simulink model "KalSim"  (Simulink 8.2)
settings: Solver=FixedStepDiscrete  StartTime=0.0  StopTime=16  FixedStep=0.005  RelTol=1e-3
PostLoadFcn:
  | , if any(exist('dsrtsu_mdlpostloadfcn', 'file') == [2, 3, 6]), try dsrtsu_mdlpostloadfcn('Execute', bdroot); catch fprintf('Error in PostLoadFcn (dsrtsu_mdlpostloadfcn) for model "%s":\n %s\n', bdroot, lasterr); end, end,
values from neighbouring files (symbols this model uses):
  C_TASK_5MS_S = (	C_TICK_TIME_S      	)    [hcu_local_hdr.m]
  FALSE = boolean( 0 )    [hcu_local_hdr.m]
  TRUE = boolean( 1 )    [hcu_local_hdr.m]
undefined symbols (not defined in the file or in its folder): A_TTC, B_TTC, C_TTC, divide, Gamma_TTC, hcu_lib, KTTC_KalmanFilterCalRate_s, Q_TTC, R_TTC_Position, R_TTC_RelAccel, R_TTC_RelVelocity
libraries: dspmtrx3 x3, simulink x1, dspinverses x1
settings Model: DSRTSU_INTERNAL_RTI_VER=460  DSRTSU_INTERNAL_RTI_TYPE=rti1401  RTICANMMDATA=struct('GeneralSetupData',struct('modelroot','D:\HAITEC\SVN\trunk\ADAS_Softwares\HTDragon\software\sw_development\arch','generalsettings',struct('filesettings',struct('destfolder',struct('Name','RTICANMM_FILES','Check',1),'buildfolder',struct('Name','.','Check',1),'AbsDestfolder',struct('Name','D:\HAITEC\SVN\trunk\ADAS_Softwares\HTDragon\software\sw_development\arch\RTICANMM_FILES'),'AbsBuildfolder',struct('Name','D:\HAITEC\SVN\trunk\ADAS_Softwares\HTDragon\software\sw_development\arch'))),'options',struct('addpaths',1,'rmpaths',1,'addtrcexclusion',logical(1),'cannavigator',struct('checkmonitoring',0),'show_usrtrc',0,'use_usrtrc',0),'advanced',struct('options',[1 1 1 1 1 1 1 1 1 1 1 1 1 1 1 1 1 1 1 1 1 1 1 1 1 1 1 1 1 1 1 1 1 1 1 1 1 1 1 1 1 1 1 1 1 1 1 1 1 1 1 1 1 1 1 1 1 1 1 1 1 1 1 1 1 1 1 1 1 1 1 1 1 1 1 1 1 1 1 1 1 1 1 1 1 1 1 1 1 1 1 1 1 1 1 1 1 1 1 1]),'MPSetup',{{}},'modelname','KalSim','block','KalSim'))  DSRTSU_INTERNAL_RTIFPGA=50  Creator=14014  LastModifiedBy=14014  BufferReuse=off
settings DataIOCC: SignalLoggingSaveFormat=Dataset
settings OptimizationCC: BlockReduction=off  OptimizeBlockIOStorage=off  BufferReuse=off  ExpressionFolding=off  ExpressionDepthLimit=128  LocalBlockOutputs=off
settings DebuggingCC: InheritedTsInSrcMsg=none  ParameterPrecisionLossMsg=none  FcnCallInpInsideContextMsg=EnableAllAsError  StateNameClashWarn=none
settings HardwareCC: ProdIntDivRoundTo=Zero  ProdEndianess=BigEndian  ProdHWDeviceType=Generic->Custom  TargetIntDivRoundTo=Zero  TargetEndianess=BigEndian  TargetHWDeviceType=Generic->Custom
settings RTWCC: SystemTargetFile=rti1401.tlc  MakeCommand=make_rti  TemplateMakefile=rti1401.tmf  Description=dSPACE DS1401 Hardware Platform  ProcessScript=rti1401_make_rtw_hook
settings STFCustomTargetCC: CodeReplacementLibrary=ANSI_C  ParMdlRefBuildCompliant=on  GeneratePreprocessorConditionals=Disable all  MatFileLogging=on  SystemTargetFile=rti1401.tlc
settings GRTTargetCC: CompOptLevelCompliant=off  ConcurrentExecutionCompliant=off  ExtModeMexFile=noextcomm
settings CustomProperty: DataType=RTWOptions_EnumType_C__Program Files_dSPACE RCPHIL 2015-A_MATLAB_RTI_RTI1401_TLC_rti1401_1InitialSimState  Value=RUN
settings EnumStrPairs: String=RUN

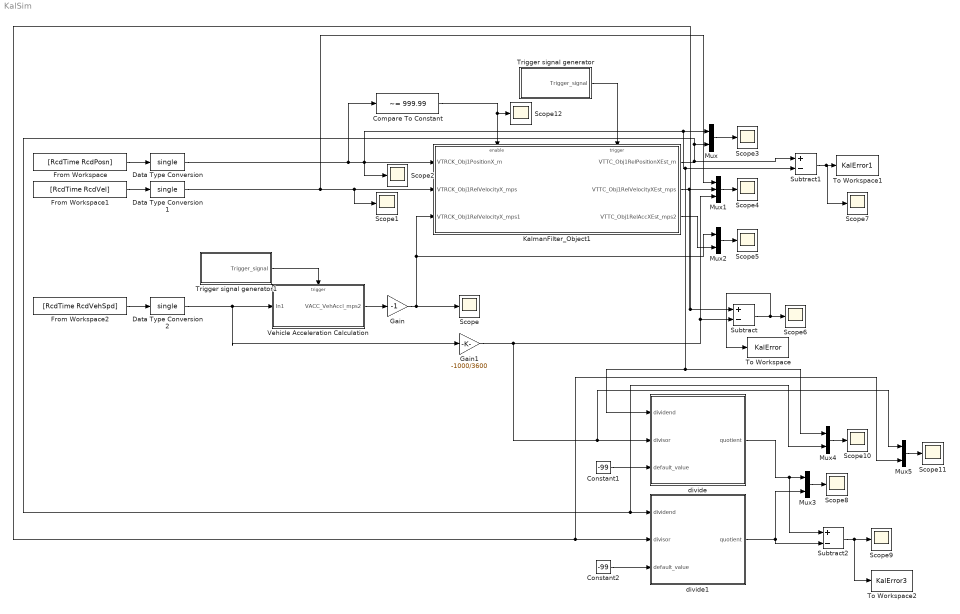
== system KalSim ==
  Compare To Constant : simulink/Logic and Bit Operations/Compare To Constant  relop=~=  const=999.99  OutDataTypeStr=boolean
  Constant1 : Constant  Value=-99  OutDataTypeStr=single
  Constant2 : Constant  Value=-99  OutDataTypeStr=single
  Data Type Conversion : DataTypeConversion  OutDataTypeStr=single
  Data Type Conversion1 : DataTypeConversion  OutDataTypeStr=single
  Data Type Conversion2 : DataTypeConversion  OutDataTypeStr=single
  From Workspace : FromWorkspace  VariableName=[RcdTime RcdPosn]
  From Workspace1 : FromWorkspace  VariableName=[RcdTime RcdVel]
  From Workspace2 : FromWorkspace  VariableName=[RcdTime RcdVehSpd]
  Gain : Gain  Gain=-1
  Gain1 : Gain  Gain=-1000/3600
  KalmanFilter_Object1 : Subsystem
  Mux{,2..5} (5 alike) : Mux  Inputs=2
  Mux1 : Mux  Inputs=3
  Scope{,1..12} (13 alike) : Scope
      Scope10 settings: SaveName=ScopeData7
      Scope11 settings: SaveName=ScopeData8
      Scope12 settings: SaveName=ScopeData9
      Scope2 settings: SaveName=ScopeData2
      Scope3 settings: SaveName=ScopeData3
      Scope4 settings: SaveName=ScopeData4
      Scope5 settings: SaveName=ScopeData5
      Scope6 settings: SaveName=KalError
      Scope7 settings: SaveName=KalError2
      Scope8 settings: SaveName=ScopeData6
      Scope9 settings: SaveName=KalError3
  Subtract : Sum  Inputs=+-
  Subtract1 : Sum  Inputs=+-
  Subtract2 : Sum  Inputs=+-
  To Workspace : ToWorkspace  VariableName=KalError  SampleTime=-1
  To Workspace1 : ToWorkspace  VariableName=KalError1  SampleTime=-1
  To Workspace2 : ToWorkspace  VariableName=KalError3  SampleTime=-1
  Trigger signal generator : Subsystem  TreatAsAtomicUnit=on
  Trigger signal generator1 : Subsystem  TreatAsAtomicUnit=on
  Vehicle Acceleration Calculation : Subsystem
  divide : Subsystem  AncestorBlock=hcu_lib/divide  RTWFcnName=divide_safe  RTWFileName=HCU_LIB  mask(divide){}
      mask help: Performs a division operation. If the divisor is found to be between -0.00001 and +0.00001 then a failsafe value is passed to the output.
      settings: RTWFcnNameOpts=User specified  RTWFileNameOpts=User specified
      mask Display: disp('Divide');
  divide1 : Subsystem  AncestorBlock=hcu_lib/divide  RTWFcnName=divide_safe  RTWFileName=HCU_LIB  mask(divide){}
      mask help: Performs a division operation. If the divisor is found to be between -0.00001 and +0.00001 then a failsafe value is passed to the output.
      settings: RTWFcnNameOpts=User specified  RTWFileNameOpts=User specified
      mask Display: disp('Divide');
  wires:
  From Workspace/1 -> Data Type Conversion/1
  From Workspace1/1 -> Data Type Conversion1/1
  Trigger signal generator/1(Trigger_signal) -> KalmanFilter_Object1/Trigger
  Compare To Constant/1 -> Scope12/1, KalmanFilter_Object1/Enable
  From Workspace2/1 -> Data Type Conversion2/1
  Data Type Conversion/1 -> Compare To Constant/1, divide/1(dividend), Mux4/1, Subtract1/2, Mux/1, Scope2/1, KalmanFilter_Object1/1(VTRCK_Obj1PositionX_m)
  Data Type Conversion1/1 -> Mux1/1, Scope1/1, KalmanFilter_Object1/2(VTRCK_Obj1RelVelocityX_mps)
  Trigger signal generator1/1(Trigger_signal) -> Vehicle Acceleration Calculation/Trigger
  Data Type Conversion2/1 -> Gain1/1, Vehicle Acceleration Calculation/1(In1)
  Vehicle Acceleration Calculation/1(VACC_VehAccl_mps2) -> Gain/1
  Gain/1 -> Scope/1, KalmanFilter_Object1/3(VTRCK_Obj1RelVelocityX_mps1), Mux2/1
  KalmanFilter_Object1/1(VTTC_Obj1RelPositionXEst_m) -> Mux4/2, divide1/1(dividend), Mux/2, Subtract1/1
  Mux/1 -> Scope3/1
  KalmanFilter_Object1/2(VTTC_Obj1RelVelocityXEst_mps) -> Mux5/2, divide1/2(divisor), Subtract/1, Mux1/2
  Mux1/1 -> Scope4/1
  Mux2/1 -> Scope5/1
  KalmanFilter_Object1/3(VTTC_Obj1RelAccXEst_mps2) -> Mux2/2
  Gain1/1 -> Mux5/1, divide/2(divisor), Subtract/2, Mux1/3
  Subtract/1 -> To Workspace/1, Scope6/1
  Subtract1/1 -> Scope7/1, To Workspace1/1
  Constant1/1 -> divide/3(default_value)
  Constant2/1 -> divide1/3(default_value)
  Mux3/1 -> Scope8/1
  divide/1(quotient) -> Subtract2/1, Mux3/1
  divide1/1(quotient) -> Subtract2/2, Mux3/2
  Subtract2/1 -> To Workspace2/1, Scope9/1
  Mux4/1 -> Scope10/1
  Mux5/1 -> Scope11/1

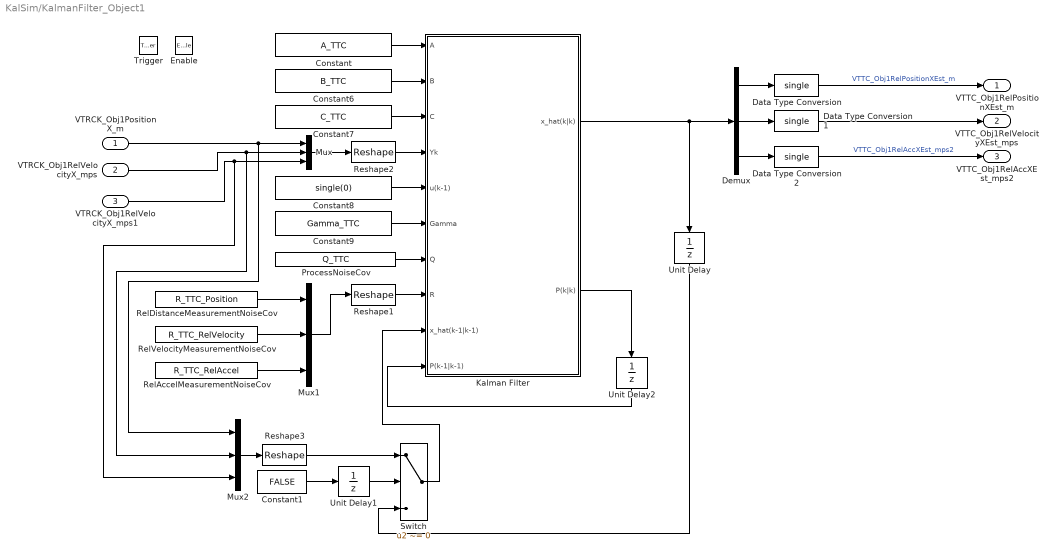
== system KalSim/KalmanFilter_Object1 ==
  VTRCK_Obj1PositionX_m : Inport
  VTRCK_Obj1RelVelocityX_mps : Inport  Port=2
  VTRCK_Obj1RelVelocityX_mps1 : Inport  Port=3
  Enable : EnablePort  StatesWhenEnabling=reset
  Trigger : TriggerPort  PortDimensions=1
  Constant : Constant  Value=A_TTC
  Constant1 : Constant  Value=FALSE
  Constant6 : Constant  Value=B_TTC
  Constant7 : Constant  Value=C_TTC
  Constant8 : Constant  Value=single(0)
  Constant9 : Constant  Value=Gamma_TTC
  Data Type Conversion : DataTypeConversion  OutDataTypeStr=single
  Data Type Conversion1 : DataTypeConversion  OutDataTypeStr=single
  Data Type Conversion2 : DataTypeConversion  OutDataTypeStr=single
  Demux : Demux  Outputs=3
  Kalman Filter : Subsystem
  Mux : Mux  Inputs=3
  Mux1 : Mux  Inputs=3
  Mux2 : Mux  Inputs=3
  ProcessNoiseCov : Constant  Value=Q_TTC
  RelAccelMeasurementNoiseCov : Constant  Value=R_TTC_RelAccel  OutDataTypeStr=single
  RelDistanceMeasurementNoiseCov : Constant  Value=R_TTC_Position  OutDataTypeStr=single
  RelVelocityMeasurementNoiseCov : Constant  Value=R_TTC_RelVelocity  OutDataTypeStr=single
  Reshape1 : Reshape  OutputDimensionality=Customize  OutputDimensions=[3,3]
  Reshape2 : Reshape  OutputDimensionality=Customize  OutputDimensions=[3,1]
  Reshape3 : Reshape  OutputDimensionality=Customize  OutputDimensions=[3,1]
  Switch : Switch  Criteria=u2 ~= 0
  Unit Delay : UnitDelay  InitialCondition=single([0;0;0])  SampleTime=-1
  Unit Delay1 : UnitDelay  InitialCondition=TRUE  SampleTime=-1
  Unit Delay2 : UnitDelay  InitialCondition=single(eye(3,3))  SampleTime=-1
  VTTC_Obj1RelPositionXEst_m : Outport  OutputWhenDisabled=reset  InitialOutput=[0]
  VTTC_Obj1RelVelocityXEst_mps : Outport  Port=2  OutputWhenDisabled=reset  InitialOutput=[0]
  VTTC_Obj1RelAccXEst_mps2 : Outport  Port=3  OutputWhenDisabled=reset  InitialOutput=[0]
  wires:
  Data Type Conversion2/1 -> VTTC_Obj1RelAccXEst_mps2/1  "VTTC_Obj1RelAccXEst_mps2"
  Data Type Conversion1/1 -> VTTC_Obj1RelVelocityXEst_mps/1
  Data Type Conversion/1 -> VTTC_Obj1RelPositionXEst_m/1  "VTTC_Obj1RelPositionXEst_m"
  Kalman Filter/2(P(k|k)) -> Unit Delay2/1
  Unit Delay2/1 -> Kalman Filter/10(P(k-1|k-1))
  Kalman Filter/1(x_hat(k|k)) -> Unit Delay/1, Demux/1
  Unit Delay/1 -> Switch/3
  Constant9/1 -> Kalman Filter/6(Gamma)
  ProcessNoiseCov/1 -> Kalman Filter/7(Q)
  Mux1/1 -> Reshape1/1
  Reshape2/1 -> Kalman Filter/4(Yk)
  Mux/1 -> Reshape2/1
  Constant8/1 -> Kalman Filter/5(u(k-1))
  Constant/1 -> Kalman Filter/1(A)
  Constant6/1 -> Kalman Filter/2(B)
  Constant7/1 -> Kalman Filter/3(C)
  RelDistanceMeasurementNoiseCov/1 -> Mux1/1
  RelVelocityMeasurementNoiseCov/1 -> Mux1/2
  Reshape1/1 -> Kalman Filter/8(R)
  VTRCK_Obj1RelVelocityX_mps/1 -> Mux2/2, Mux/2
  VTRCK_Obj1PositionX_m/1 -> Mux2/1, Mux/1
  Demux/2 -> Data Type Conversion1/1
  Demux/1 -> Data Type Conversion/1
  Demux/3 -> Data Type Conversion2/1
  Constant1/1 -> Unit Delay1/1
  Unit Delay1/1 -> Switch/2
  VTRCK_Obj1RelVelocityX_mps1/1 -> Mux2/3, Mux/3
  Mux2/1 -> Reshape3/1
  Reshape3/1 -> Switch/1
  Switch/1 -> Kalman Filter/9(x_hat(k-1|k-1))
  RelAccelMeasurementNoiseCov/1 -> Mux1/3

== system KalSim/Trigger signal generator ==
  Constant3 : Constant  Value=KTTC_KalmanFilterCalRate_s
  trigger signal generator : Subsystem  TreatAsAtomicUnit=on
  Trigger_signal : Outport
  wires:
  trigger signal generator/1(Trigger_signal) -> Trigger_signal/1
  Constant3/1 -> trigger signal generator/1(Time_dur [s])

== system KalSim/Trigger signal generator1 ==
  Constant3 : Constant  Value=0.05
  trigger signal generator : Subsystem  TreatAsAtomicUnit=on
  Trigger_signal : Outport
  wires:
  trigger signal generator/1(Trigger_signal) -> Trigger_signal/1
  Constant3/1 -> trigger signal generator/1(Time_dur [s])

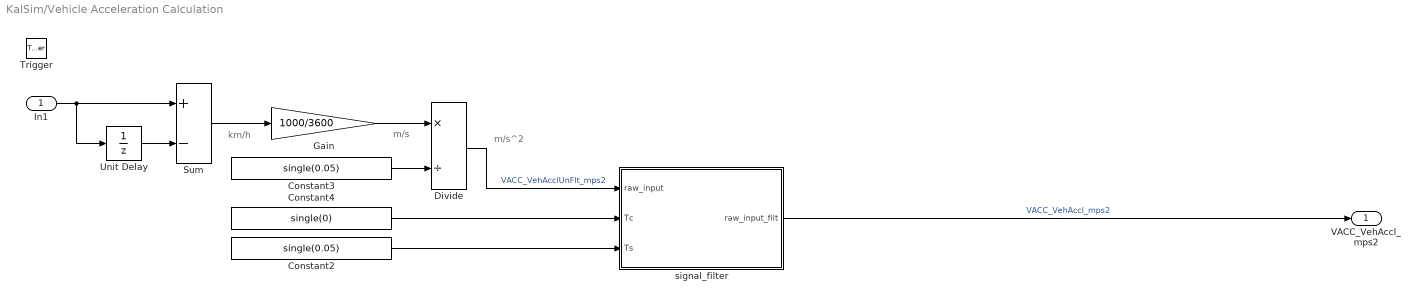
== system KalSim/Vehicle Acceleration Calculation ==
  note: m/s^2
  note: m/s
  note: km/h
  In1 : Inport
  Trigger : TriggerPort
  Constant2 : Constant  Value=single(0.05)
  Constant3 : Constant  Value=single(0.05)
  Constant4 : Constant  Value=single(0)
  Divide : Product  Inputs=*/
  Gain : Gain  Gain=1000/3600
  Sum : Sum  Inputs=+-
  Unit Delay : UnitDelay  SampleTime=-1
  signal_filter : Subsystem
  VACC_VehAccl_mps2 : Outport
  wires:
  signal_filter/1(raw_input_filt) -> VACC_VehAccl_mps2/1  "VACC_VehAccl_mps2"
  Constant3/1 -> Divide/2
  Gain/1 -> Divide/1
  Sum/1 -> Gain/1
  Unit Delay/1 -> Sum/2
  In1/1 -> Sum/1, Unit Delay/1
  Constant2/1 -> signal_filter/3(Ts)
  Constant4/1 -> signal_filter/2(Tc)
  Divide/1 -> signal_filter/1(raw_input)  "VACC_VehAcclUnFlt_mps2"

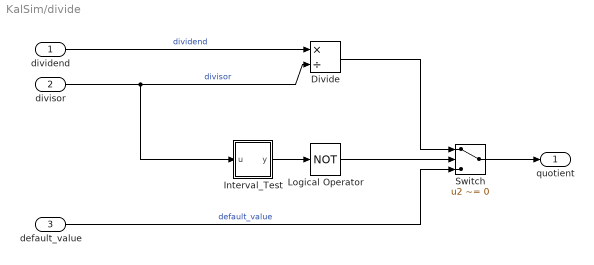
== system KalSim/divide ==
  dividend : Inport
  divisor : Inport  Port=2
  default_value : Inport  Port=3
  Divide : Product  Inputs=*/
  Interval_Test : Subsystem  mask(Interval Test){IntervalClosedRight=on, uplimit=1, IntervalClosedLeft=on, lowlimit=-1, LogicOutDataTypeMode=boolean}
      mask prompts: IntervalClosedRight "Interval closed on right"; uplimit "Upper limit:"; IntervalClosedLeft "Interval closed on left"; lowlimit "Lower limit:"; LogicOutDataTypeMode "Output data type mode:"
      mask help: If the input is in the interval between the lower limit and the upper limit, then the output is TRUE, otherwise it is FALSE.
      mask init:
      | if IntervalClosedLeft
      |   lOff = 0;
      |   lRelop = '<=';
      | else
      |   lOff = 0.1;
      |   lRelop = '<';
      | end
      | if IntervalClosedRight
      |   rOff = 0;
      |   uRelop = '<=';
      | else
      |   rOff = 0.1;
      |   uRelop = '<';
      | end
      | 
      | blkH = gcbh;
      | blkName = getfullname(blkH);
      | 
      | set_param([blkName,'/Upper Test'],'relop',uRelop);
      | set_param([blkName,'/Lower Test'],'relop',lRelop);
      | if strcmp(get_param(blkH,'LogicOutDataTypeMode'),'boolean')
      | set_param([blkName,'/AND'],'OutDataTypeMode','Boolean');
      | else
      | set_param([blkName,'/AND'],'OutDataTypeMode','Specify via dialog');
      | end
      mask TypeOptions LogicOutDataTypeMode: uint8 | boolean
      mask Display: plot([0 1],[0.3 0.3],[0.3 0.3],[0 1],[0 0.2 0.2],[0.35 0.35 0.55-lOff],[0.2 0.2 0.55 0.55],[0.55+lOff 0.75 0.75 0.55+rOff],[0.55 0.55 1],[0.55-rOff 0.35 0.35]);
  Logical Operator : Logic  Operator=NOT  Inputs=1  AllPortsSameDT=off  OutDataTypeStr=boolean
  Switch : Switch  Criteria=u2 ~= 0  Threshold=0.5
  quotient : Outport
  wires:
  dividend/1 -> Divide/1  "dividend"
  divisor/1 -> Divide/2, Interval_Test/1(u)  "divisor"
  Divide/1 -> Switch/1
  Switch/1 -> quotient/1
  Interval_Test/1(y) -> Logical Operator/1
  default_value/1 -> Switch/3  "default_value"
  Logical Operator/1 -> Switch/2

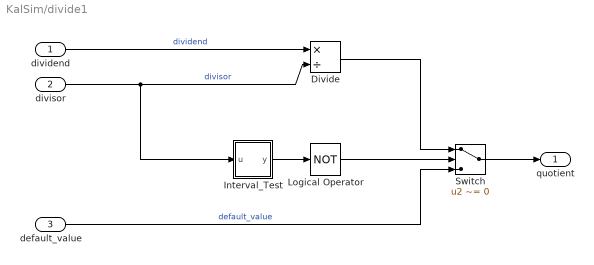
== system KalSim/divide1 ==
  dividend : Inport
  divisor : Inport  Port=2
  default_value : Inport  Port=3
  Divide : Product  Inputs=*/
  Interval_Test : Subsystem  mask(Interval Test){IntervalClosedRight=on, uplimit=1, IntervalClosedLeft=on, lowlimit=-1, LogicOutDataTypeMode=boolean}
      mask prompts: IntervalClosedRight "Interval closed on right"; uplimit "Upper limit:"; IntervalClosedLeft "Interval closed on left"; lowlimit "Lower limit:"; LogicOutDataTypeMode "Output data type mode:"
      mask help: If the input is in the interval between the lower limit and the upper limit, then the output is TRUE, otherwise it is FALSE.
      mask init: same as KalSim/divide/Interval_Test
      mask TypeOptions LogicOutDataTypeMode: uint8 | boolean
      mask Display: plot([0 1],[0.3 0.3],[0.3 0.3],[0 1],[0 0.2 0.2],[0.35 0.35 0.55-lOff],[0.2 0.2 0.55 0.55],[0.55+lOff 0.75 0.75 0.55+rOff],[0.55 0.55 1],[0.55-rOff 0.35 0.35]);
  Logical Operator : Logic  Operator=NOT  Inputs=1  AllPortsSameDT=off  OutDataTypeStr=boolean
  Switch : Switch  Criteria=u2 ~= 0  Threshold=0.5
  quotient : Outport
  wires:
  Logical Operator/1 -> Switch/2
  default_value/1 -> Switch/3  "default_value"
  Interval_Test/1(y) -> Logical Operator/1
  Switch/1 -> quotient/1
  Divide/1 -> Switch/1
  divisor/1 -> Interval_Test/1(u), Divide/2  "divisor"
  dividend/1 -> Divide/1  "dividend"

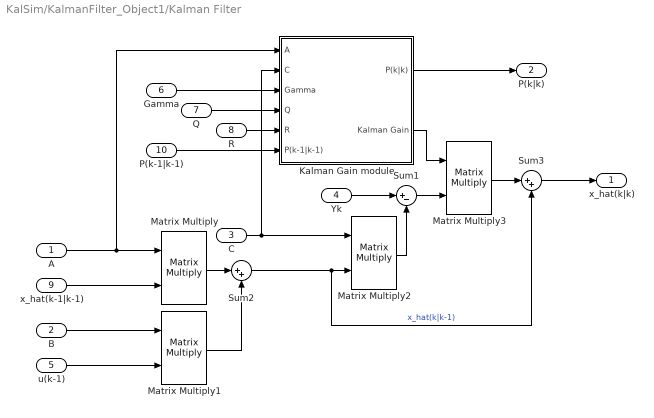
== system KalSim/KalmanFilter_Object1/Kalman Filter ==
  A : Inport
  B : Inport  Port=2
  C : Inport  Port=3
  Yk : Inport  Port=4
  u(k-1) : Inport  Port=5
  Gamma : Inport  Port=6
  Q : Inport  Port=7
  R : Inport  Port=8
  x_hat(k-1|k-1) : Inport  Port=9
  P(k-1|k-1) : Inport  Port=10
  Kalman Gain module : Subsystem
  Matrix Multiply{,1..3} (4 alike) : Product  Multiplication=Matrix(*)
  Sum1 : Sum  Inputs=|+-
  Sum2 : Sum  Inputs=|++
  Sum3 : Sum  Inputs=|++
  x_hat(k|k) : Outport
  P(k|k) : Outport  Port=2
  wires:
  A/1 -> Matrix Multiply/1, Kalman Gain module/1(A)
  x_hat(k-1|k-1)/1 -> Matrix Multiply/2
  Matrix Multiply/1 -> Sum2/1
  B/1 -> Matrix Multiply1/1
  u(k-1)/1 -> Matrix Multiply1/2
  Matrix Multiply1/1 -> Sum2/2
  Yk/1 -> Sum1/1
  C/1 -> Matrix Multiply2/1, Kalman Gain module/2(C)
  Sum2/1 -> Matrix Multiply2/2, Sum3/2  "x_hat(k|k-1)"
  Matrix Multiply2/1 -> Sum1/2
  Kalman Gain module/2(Kalman Gain) -> Matrix Multiply3/1
  Sum1/1 -> Matrix Multiply3/2
  Matrix Multiply3/1 -> Sum3/1
  Sum3/1 -> x_hat(k|k)/1
  Gamma/1 -> Kalman Gain module/3(Gamma)
  Q/1 -> Kalman Gain module/4(Q)
  R/1 -> Kalman Gain module/5(R)
  Kalman Gain module/1(P(k|k)) -> P(k|k)/1
  P(k-1|k-1)/1 -> Kalman Gain module/6(P(k-1|k-1))

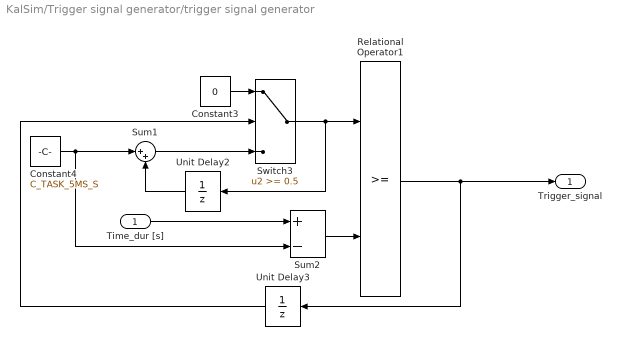
== system KalSim/Trigger signal generator/trigger signal generator ==
  Time_dur [s] : Inport
  Constant3 : Constant  Value=0  OutDataTypeStr=single
  Constant4 : Constant  Value=C_TASK_5MS_S
  Relational Operator1 : RelationalOperator  OutDataTypeStr=boolean
  Sum1 : Sum  Inputs=|++  SaturateOnIntegerOverflow=on  InputSameDT=on
  Sum2 : Sum  Inputs=+-
  Switch3 : Switch  Threshold=0.5
  Unit Delay2 : UnitDelay  SampleTime=-1
  Unit Delay3 : UnitDelay  SampleTime=-1
  Trigger_signal : Outport  OutputWhenDisabled=reset  InitialOutput=[0]
  wires:
  Sum2/1 -> Relational Operator1/2
  Unit Delay3/1 -> Switch3/2
  Unit Delay2/1 -> Sum1/2
  Switch3/1 -> Relational Operator1/1, Unit Delay2/1
  Constant3/1 -> Switch3/1
  Time_dur [s]/1 -> Sum2/1
  Relational Operator1/1 -> Unit Delay3/1, Trigger_signal/1
  Constant4/1 -> Sum2/2, Sum1/1
  Sum1/1 -> Switch3/3

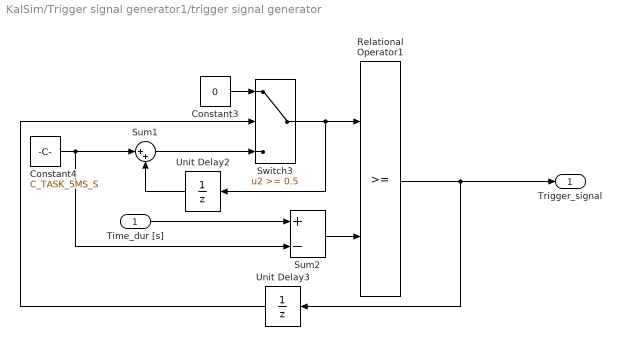
== system KalSim/Trigger signal generator1/trigger signal generator ==
  Time_dur [s] : Inport
  Constant3 : Constant  Value=0  OutDataTypeStr=single
  Constant4 : Constant  Value=C_TASK_5MS_S
  Relational Operator1 : RelationalOperator  OutDataTypeStr=boolean
  Sum1 : Sum  Inputs=|++  SaturateOnIntegerOverflow=on  InputSameDT=on
  Sum2 : Sum  Inputs=+-
  Switch3 : Switch  Threshold=0.5
  Unit Delay2 : UnitDelay  SampleTime=-1
  Unit Delay3 : UnitDelay  SampleTime=-1
  Trigger_signal : Outport  OutputWhenDisabled=reset  InitialOutput=[0]
  wires:
  Sum2/1 -> Relational Operator1/2
  Unit Delay3/1 -> Switch3/2
  Unit Delay2/1 -> Sum1/2
  Switch3/1 -> Relational Operator1/1, Unit Delay2/1
  Constant3/1 -> Switch3/1
  Time_dur [s]/1 -> Sum2/1
  Relational Operator1/1 -> Unit Delay3/1, Trigger_signal/1
  Constant4/1 -> Sum2/2, Sum1/1
  Sum1/1 -> Switch3/3

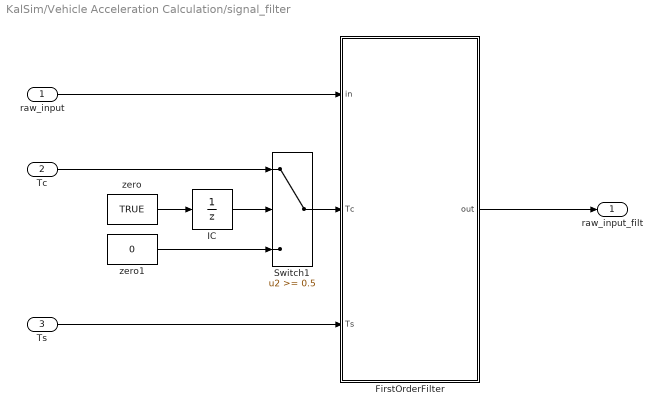
== system KalSim/Vehicle Acceleration Calculation/signal_filter ==
  raw_input : Inport
  Tc : Inport  Port=2
  Ts : Inport  Port=3
  FirstOrderFilter : Subsystem  RTWFileName=HCU_LIB
      settings: RTWFileNameOpts=User specified
  IC : UnitDelay  Tag=struct('comment',struct('text','','placement',1),'logdata',struct('maxnumvals',inf,'plotchannels',[],'stepsize',0,'downsampling',1,'loggingmode',3,'channels',1),'output',struct('width',1,'name','$S_$B','unit','','type','Int16','offset',0,'max',NaN,'min',NaN,'freeze',1,'lsb',1,'arb',0,'class','default','address','','description','','autoscalingmode',1,'lowerheadroom',1,'upperheadroom',1,'headroomunit','bit','checkmin',0,'checkmax',0,'show',0,'initial','2'),'state',0,'dt','-1','date',731455.586925799)  SampleTime=-1
  Switch1 : Switch  Tag=struct('comment',struct('text','','placement',1),'logdata',struct('maxnumvals',inf,'plotchannels',[],'stepsize',0,'downsampling',1,'loggingmode',3,'channels',1),'output',struct('width',1,'name','$S_$B','unit','','type','Int32Bin15','offset',0,'max',65535,'min',-65536,'freeze',1,'lsb',2^-15,'arb',0,'class','default','address','','description','','autoscalingmode',1,'lowerheadroom',1,'upperheadroom',1,'headroomunit','bit','checkmin',0,'checkmax',0,'show',0),'threshold',struct('width',1,'name','$S_$B_threshold','unit','','type','Int16','offset',0,'max',NaN,'min',NaN,'freeze',1,'lsb',1,'arb',0,'class','default','address','','description','','value','1','scalar',0),'date',731455.58657044)  Threshold=0.5  InputSameDT=on
  zero : Constant  Tag=struct('comment',struct('text','','placement',1),'output',struct('width',1,'name','$S_$B','unit','','type','Int16','offset',0,'max',NaN,'min',NaN,'freeze',1,'lsb',1,'arb',0,'class','default','address','','description','','value','0','tolerance',1,'show',0),'date',731455.58675544)  Value=TRUE
  zero1 : Constant  Tag=struct('comment',struct('text','','placement',1),'output',struct('width',1,'name','$S_$B','unit','','type','Int16','offset',0,'max',NaN,'min',NaN,'freeze',1,'lsb',1,'arb',0,'class','default','address','','description','','value','0','tolerance',1,'show',0),'date',731455.58675544)  Value=0  OutDataTypeStr=single
  raw_input_filt : Outport
  wires:
  zero/1 -> IC/1
  raw_input/1 -> FirstOrderFilter/1(in)
  Tc/1 -> Switch1/1
  Ts/1 -> FirstOrderFilter/3(Ts)
  IC/1 -> Switch1/2
  FirstOrderFilter/1(out) -> raw_input_filt/1
  Switch1/1 -> FirstOrderFilter/2(Tc)
  zero1/1 -> Switch1/3

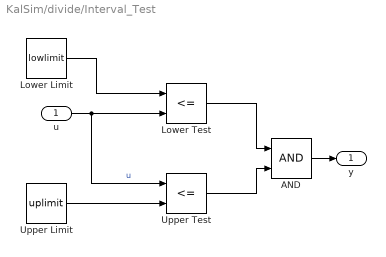
== system KalSim/divide/Interval_Test ==
  u : Inport
  AND : Logic  AllPortsSameDT=off  OutDataTypeStr=boolean
  Lower Limit : Constant  DisableCoverage=on  Value=lowlimit  OutDataTypeStr=Inherit: Inherit via back propagation
  Lower Test : RelationalOperator  DisableCoverage=on  Operator=<=  OutDataTypeStr=boolean  ZeroCross=off
  Upper Limit : Constant  DisableCoverage=on  Value=uplimit  OutDataTypeStr=Inherit: Inherit via back propagation
  Upper Test : RelationalOperator  DisableCoverage=on  Operator=<=  OutDataTypeStr=boolean  ZeroCross=off
  y : Outport
  wires:
  Lower Limit/1 -> Lower Test/1
  Upper Limit/1 -> Upper Test/2
  Lower Test/1 -> AND/1
  Upper Test/1 -> AND/2
  u/1 -> Lower Test/2, Upper Test/1  "u"
  AND/1 -> y/1

== system KalSim/divide1/Interval_Test ==
  u : Inport
  AND : Logic  AllPortsSameDT=off  OutDataTypeStr=boolean
  Lower Limit : Constant  DisableCoverage=on  Value=lowlimit  OutDataTypeStr=Inherit: Inherit via back propagation
  Lower Test : RelationalOperator  DisableCoverage=on  Operator=<=  OutDataTypeStr=boolean  ZeroCross=off
  Upper Limit : Constant  DisableCoverage=on  Value=uplimit  OutDataTypeStr=Inherit: Inherit via back propagation
  Upper Test : RelationalOperator  DisableCoverage=on  Operator=<=  OutDataTypeStr=boolean  ZeroCross=off
  y : Outport
  wires:
  AND/1 -> y/1
  u/1 -> Upper Test/1, Lower Test/2  "u"
  Upper Test/1 -> AND/2
  Lower Test/1 -> AND/1
  Upper Limit/1 -> Upper Test/2
  Lower Limit/1 -> Lower Test/1

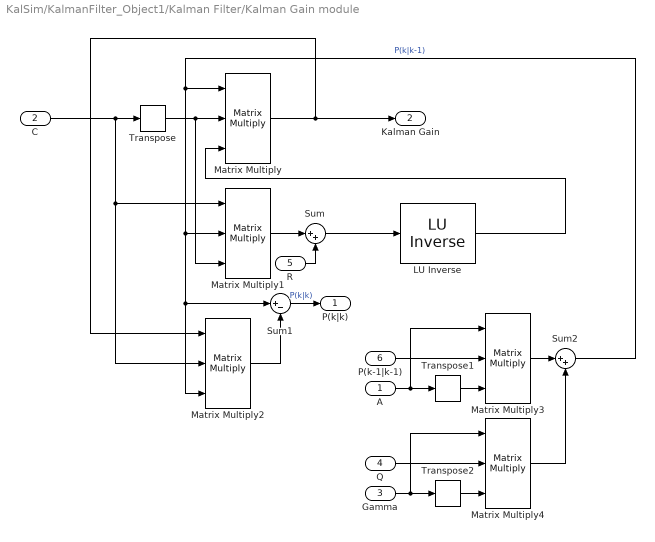
== system KalSim/KalmanFilter_Object1/Kalman Filter/Kalman Gain module ==
  A : Inport
  C : Inport  Port=2
  Gamma : Inport  Port=3
  Q : Inport  Port=4
  R : Inport  Port=5
  P(k-1|k-1) : Inport  Port=6
  " LU Inverse" : dspinverses/ LU Inverse
  Matrix Multiply{,1..4} (5 alike) : Product  Inputs=3  Multiplication=Matrix(*)
  Sum : Sum  Inputs=|++
  Sum1 : Sum  Inputs=|+-
  Sum2 : Sum  Inputs=|++
  Transpose : dspmtrx3/Transpose  Hermitian=off  overflowFlag=on
  Transpose1 : dspmtrx3/Transpose  Hermitian=off  overflowFlag=on
  Transpose2 : dspmtrx3/Transpose  Hermitian=off  overflowFlag=on
  P(k|k) : Outport
  Kalman Gain : Outport  Port=2
  wires:
  C/1 -> Transpose/1, Matrix Multiply1/1, Matrix Multiply2/2
  Transpose/1 -> Matrix Multiply/2, Matrix Multiply1/3
  Matrix Multiply1/1 -> Sum/1
  R/1 -> Sum/2
  Sum/1 -> " LU Inverse"/1
  " LU Inverse"/1 -> Matrix Multiply/3
  Matrix Multiply/1 -> Matrix Multiply2/1, Kalman Gain/1
  Matrix Multiply2/1 -> Sum1/2
  A/1 -> Transpose1/1, Matrix Multiply3/1
  Transpose1/1 -> Matrix Multiply3/3
  Matrix Multiply3/1 -> Sum2/1
  Transpose2/1 -> Matrix Multiply4/3
  Gamma/1 -> Transpose2/1, Matrix Multiply4/1
  Q/1 -> Matrix Multiply4/2
  Matrix Multiply4/1 -> Sum2/2
  Sum2/1 -> Matrix Multiply/1, Matrix Multiply1/2, Sum1/1, Matrix Multiply2/3  "P(k|k-1)"
  P(k-1|k-1)/1 -> Matrix Multiply3/2
  Sum1/1 -> P(k|k)/1  "P(k|k)"

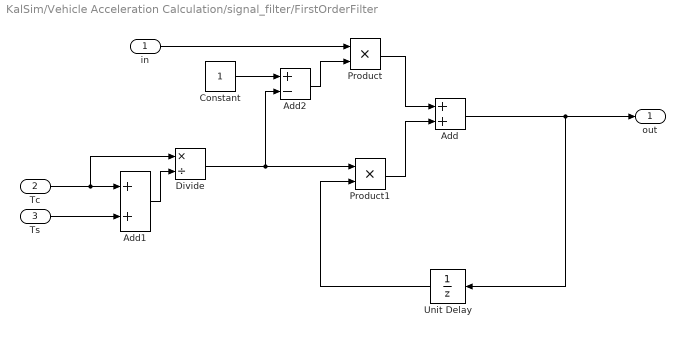
== system KalSim/Vehicle Acceleration Calculation/signal_filter/FirstOrderFilter ==
  in : Inport
  Tc : Inport  Port=2
  Ts : Inport  Port=3
  Add : Sum
  Add1 : Sum
  Add2 : Sum  Inputs=+-
  Constant : Constant  OutDataTypeStr=single
  Divide : Product  Inputs=*/
  Product : Product  RndMeth=Zero
  Product1 : Product  RndMeth=Zero
  Unit Delay : UnitDelay  SampleTime=-1
  out : Outport
  wires:
  Add/1 -> Unit Delay/1, out/1
  Product1/1 -> Add/2
  Product/1 -> Add/1
  Add2/1 -> Product/2
  in/1 -> Product/1
  Divide/1 -> Product1/1, Add2/2
  Constant/1 -> Add2/1
  Add1/1 -> Divide/2
  Ts/1 -> Add1/2
  Tc/1 -> Divide/1, Add1/1
  Unit Delay/1 -> Product1/2
